simulink model "CuantUnifSin"  (R2017b)
settings: Solver=ode45  StartTime=0.0  StopTime=10.0  RelTol=1e-3  EnableMultiTasking=on
values from neighbouring files (symbols this model uses):
  n = N(i)    [CuantNoUniformeVoz.m]    (also in CuantUniformeSeno.m; CuantUniformeVoz.m)
settings Model: Creator=Jorge Armando  LastModifiedBy=adgp97
settings DataIOCC: SaveFormat=Array
settings OptimizationCC: LifeSpan=inf
settings DebuggingCC: UnderspecifiedInitializationDetection=Classic  MergeDetectMultiDrivingBlocksExec=none  SolverPrmCheckMsg=warning  StateNameClashWarn=warning  SFUnexpectedBacktrackingDiag=warning  SFNoUnconditionalDefaultTransitionDiag=warning  SFExecutionAtInitializationDiag=none
settings HardwareCC: ProdBitPerPointer=32  ProdBitPerSizeT=32  ProdBitPerPtrDiffT=32  ProdLargestAtomicFloat=None  ProdIntDivRoundTo=Undefined  ProdEndianess=Unspecified  ProdWordSize=32  ProdHWDeviceType=32-bit Generic
settings ModelReferenceCC: PropagateSignalLabelsOutOfModel=off
settings CodeAppCC: StateflowObjectComments=on
settings GRTTargetCC: TargetLangStandard=C89/C90 (ANSI)  GeneratePreprocessorConditionals=Disable all
settings ConfigComp: CovMetricSettings=dw  CovHtmlReporting=on  CovSaveCumulativeToWorkspaceVar=on  CovSaveSingleToWorkspaceVar=on  CovExternalEMLEnable=off  CovSFcnEnable=off

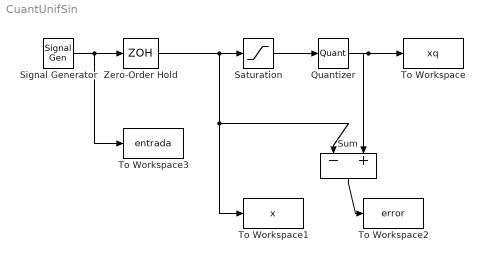
== system CuantUnifSin ==
  Quantizer : Quantizer  QuantizationInterval=2^(1-n)
  Saturation : Saturate  UpperLimit=1  LowerLimit=-1
  Signal Generator : SignalGenerator
  Sum : Sum  Inputs=|-+
  To Workspace : ToWorkspace  VariableName=xq  SampleTime=-1
  To Workspace1 : ToWorkspace  VariableName=x  SampleTime=-1
  To Workspace2 : ToWorkspace  VariableName=error  SampleTime=-1
  To Workspace3 : ToWorkspace  VariableName=entrada  SampleTime=-1
  Zero-Order Hold : ZeroOrderHold  SampleTime=1/100
  wires:
  Signal Generator/1 -> To Workspace3/1, Zero-Order Hold/1
  Zero-Order Hold/1 -> To Workspace1/1, Sum/1, Saturation/1
  Saturation/1 -> Quantizer/1
  Quantizer/1 -> To Workspace/1, Sum/2
  Sum/1 -> To Workspace2/1
